simulink model "system_identification_good"  (R2024a)
settings: Solver=ode4  StartTime=0.0  StopTime=inf  FixedStep=0.002  RelTol=1e-3  EnableMultiTasking=on
undefined symbols (not defined in the file or in its folder): HIL
libraries: quarc_library x6
settings Model: ExtModeTrigDuration=10000  Creator=brusie  LastModifiedBy=brusie
settings SolverCC: AlgebraicLoopSolver=TrustRegion  PositivePriorityOrder=on
settings DataIOCC: ReturnWorkspaceOutputs=off
settings DebuggingCC: UnconnectedInputMsg=warning  UnconnectedOutputMsg=warning  UnconnectedLineMsg=warning  ArithmeticOperatorsInVariantConditions=warning
settings ModelReferenceCC: EnableRefExpFcnMdlSchedulingChecks=on
settings SFSimCC: SimUseLocalCustomCode=off  CustomCodeUndefinedFunction=UseInterfaceOnly
settings RTWCC: Description=QUARC Win64 Target Using Toolchain  SystemTargetFile=quarc_win64.tlc  TemplateMakefile=quarc_default_tmf  RTWUseLocalCustomCode=off  Toolchain=QUARC win64 | nmake (64-bit Windows)  BuildConfiguration=Faster Runs  GPUComputeCapability=3.5
settings CodeAppCC: StateflowObjectComments=on
settings STFCustomTargetCC: ConcurrentExecutionCompliant=on  SystemTargetFile=quarc_win64.tlc
settings GRTTargetCC: ParMdlRefBuildCompliant=off  CompOptLevelCompliant=off  CombineOutputUpdateFcns=off  MatFileLogging=off  CPPClassGenCompliant=off  GRTInterface=on  ExtMode=on  ExtModeMexFile=quarc_comm
settings ConfigComp: CovMetricSettings=dswe

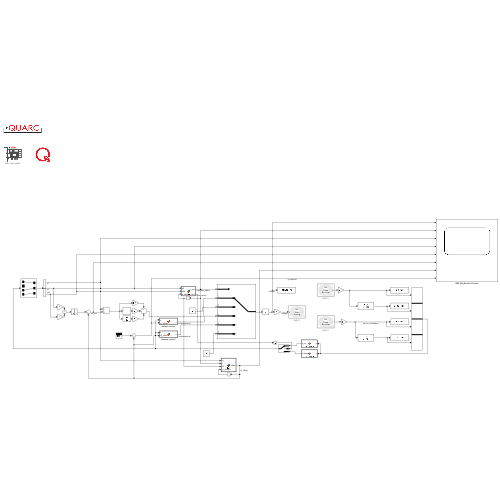
[thumbnail: Simulink's stored preview of the top-level diagram]
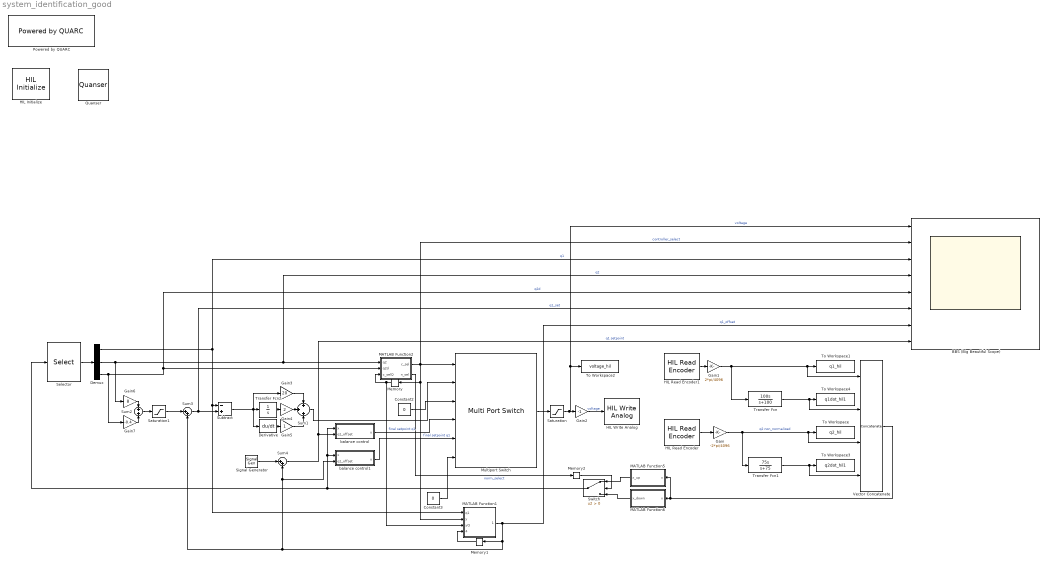
== system system_identification_good ==
  BBS (Big Beautiful Scope) : Scope  NumInputPorts=8
  Constant2 : Constant  Value=0
  Constant3 : Constant  Value=0
  Demux : Demux  Outputs=3
      settings: DisplayOption=none
  Derivative : Derivative
  Gain : Gain  Gain=-2*pi/4096
  Gain1 : Gain  Gain=2*pi/4096
  Gain2 : Gain  Gain=-1
  Gain3 : Gain  Gain=20
  Gain4 : Gain  Gain=2
  Gain5 : Gain
  Gain6 : Gain  Gain=8
  Gain7 : Gain  Gain=-0.4
  HIL Initialize : quarc_library/Data Acquisition/Generic/Configuration/HIL Initialize  object_name=HIL-1  board_type=q2_usb  board_number=0  board_options=d0=digital;d1=digital;led=auto;update_rate=normal;decimation=1  exclusive=off  active=on  hardware_clocks=[0]  clock_modes=[]  initial_clock_frequencies=[]  set_clock_params_at_start=off  set_clock_params_at_switch_in=off  set_clock_frequencies_at_start=off  set_clock_frequencies_at_switch_in=off  analog_input_channels=[0:1]  analog_input_configurations=[]  analog_input_maximums=10  analog_input_minimums=-10  set_analog_input_params_at_start=on  set_analog_input_params_at_switch_in=off  analog_output_channels=[0:1]  analog_output_maximums=10  analog_output_minimums=-10  initial_analog_outputs=[0]  final_analog_outputs=[0]  watchdog_analog_outputs=0  set_analog_output_params_at_start=on  set_analog_output_params_at_switch_in=off  set_analog_outputs_at_start=on  set_analog_outputs_at_switch_in=off  set_analog_outputs_at_terminate=on  set_analog_outputs_at_switch_out=off  set_analog_outputs_on_watchdog=off  digital_input_channels=[]  digital_output_channels=[]  digital_output_configuration=[]  initial_digital_outputs=[1]  final_digital_outputs=[1]  watchdog_digital_outputs=[1]  set_digital_output_params_at_start=off  set_digital_output_params_at_switch_in=off  set_digital_outputs_at_start=on  set_digital_outputs_at_switch_in=off  set_digital_outputs_at_terminate=on  set_digital_outputs_at_switch_out=off  set_digital_outputs_on_watchdog=off  encoder_channels=[0:1]  quadrature=[4]  encoder_filter_frequency=[]  initial_encoder_counts=[0]  set_encoder_params_at_start=on  set_encoder_params_at_switch_in=off  set_encoder_counts_at_start=on  set_encoder_counts_at_switch_in=off  pwm_channels=[]  pwm_modes=[0]  pwm_frequency=1/0.020  pwm_configuration=[]  pwm_alignment=[]  pwm_polarity=[]  pwm_leading_deadband=[]  pwm_trailing_deadband=[]  initial_pwm_outputs=[0]  final_pwm_outputs=[0]  watchdog_pwm_outputs=[0]  set_pwm_params_at_start=on  set_pwm_params_at_switch_in=off  set_pwm_outputs_at_start=on  set_pwm_outputs_at_switch_in=off  set_pwm_outputs_at_terminate=on  set_pwm_outputs_at_switch_out=off  set_pwm_outputs_on_watchdog=off  other_output_channels=[]  initial_other_outputs=[]  final_other_outputs=[]  watchdog_other_outputs=[]  set_other_outputs_at_start=off  set_other_outputs_at_switch_in=off  set_other_outputs_at_terminate=off  set_other_outputs_at_switch_out=off  set_other_outputs_on_watchdog=off
  HIL Read Encoder : quarc_library/Data Acquisition/Generic/Immediate I//O/HIL Read Encoder  object_name=HIL-1  channels=[1]  sample_time=qc_get_step_size  active=on  vector_output=off  data_type_mode=Inherit via back propagation  data_type=double
  HIL Read Encoder1 : quarc_library/Data Acquisition/Generic/Immediate I//O/HIL Read Encoder  object_name=HIL-1  channels=0  sample_time=qc_get_step_size  active=on  vector_output=off  data_type_mode=Inherit via back propagation  data_type=double
  HIL Write Analog : quarc_library/Data Acquisition/Generic/Immediate I//O/HIL Write Analog  object_name=HIL-1  channels=0  sample_time=-1  active=off  vector_input=off
  MATLAB Function1 : MATLAB Function  TreatAsAtomicUnit=on
  MATLAB Function2 : MATLAB Function  TreatAsAtomicUnit=on
  MATLAB Function5 : MATLAB Function  TreatAsAtomicUnit=on
  MATLAB Function6 : MATLAB Function  TreatAsAtomicUnit=on
  Memory : Memory
  Memory1 : Memory
  Memory2 : Memory
  Multiport Switch : MultiPortSwitch  Inputs=4  DataPortForDefault=Additional data port  SaturateOnIntegerOverflow=off  InputSameDT=off
  Powered by QUARC : quarc_library/Logos/Powered by QUARC
  Quanser : quarc_library/Logos/Quanser
  Saturation : Saturate  UpperLimit=10  LowerLimit=-10
  Saturation1 : Saturate  UpperLimit=pi/6  LowerLimit=-pi/6
  Selector : Selector  InputPortWidth=4  IndexOptions=Index vector (dialog)  Indices=[1 3 4]  OutputSizes=1
  Signal Generator : SignalGenerator  Amplitude=0  Units=rad/sec
  Subtract : Sum  Inputs=-+
  Sum1 : Sum  Inputs=+|+|+
  Sum2 : Sum
  Sum3 : Sum  Inputs=|++
  Sum4 : Sum  Inputs=|++
  Switch : Switch  Criteria=u2 > Threshold  SaturateOnIntegerOverflow=off  InputSameDT=off
  To Workspace : ToWorkspace  VariableName=q2_hil  SaveFormat=Structure With Time  SampleTime=-1
  To Workspace1 : ToWorkspace  VariableName=q1_hil  SaveFormat=Structure With Time  SampleTime=-1
  To Workspace2 : ToWorkspace  VariableName=voltage_hil  SaveFormat=Structure With Time  SampleTime=-1
  To Workspace3 : ToWorkspace  VariableName=q2dot_hil1  SaveFormat=Structure With Time  SampleTime=-1
  To Workspace4 : ToWorkspace  VariableName=q1dot_hil1  SaveFormat=Structure With Time  SampleTime=-1
  Transfer Fcn : TransferFcn  Numerator=[100 0]  Denominator=[1 100]
  Transfer Fcn1 : TransferFcn  Numerator=[75 0]  Denominator=[1 75]
  Transfer Fcn2 : TransferFcn  Denominator=[1 0]
  Vector Concatenate : Concatenate  NumInputs=4
  balance control : MATLAB Function  TreatAsAtomicUnit=on
  balance control1 : MATLAB Function  TreatAsAtomicUnit=on
  wires:
  Saturation/1 -> To Workspace2/1, BBS (Big Beautiful Scope)/1, Gain2/1  "voltage"
  Gain1/1 -> Vector Concatenate/1, To Workspace1/1, Transfer Fcn/1
  HIL Read Encoder1/1 -> Gain1/1
  HIL Read Encoder/1 -> Gain/1
  Transfer Fcn/1 -> Vector Concatenate/2, To Workspace4/1
  Transfer Fcn1/1 -> Vector Concatenate/4, To Workspace3/1
  Constant2/1 -> Multiport Switch/3
  Derivative/1 -> Gain5/1
  Transfer Fcn2/1 -> Gain4/1
  Gain3/1 -> Sum1/1
  Gain5/1 -> Sum1/3
  Gain4/1 -> Sum1/2
  Demux/3 -> Gain7/1, MATLAB Function2/2(q2d), BBS (Big Beautiful Scope)/5  "q2d"
  Gain7/1 -> Sum2/2
  Memory/1 -> MATLAB Function2/3(c_selQ), MATLAB Function1/3(yQ)
  Multiport Switch/1 -> Saturation/1
  Gain6/1 -> Sum2/1
  Gain/1 -> Vector Concatenate/3, To Workspace/1, Transfer Fcn1/1  "q2 non_normalized"
  Demux/1 -> BBS (Big Beautiful Scope)/3, MATLAB Function1/1(q1), Subtract/1  "q1"
  Selector/1 -> Demux/1
  Gain2/1 -> HIL Write Analog/1  "voltage"
  MATLAB Function1/1(q1_offset) -> Sum3/2, balance control1/2(q1_offset), Sum4/2, Memory1/1, BBS (Big Beautiful Scope)/7  "q1_offset"
  Memory1/1 -> MATLAB Function1/4(q1_offsetQ)
  Sum2/1 -> Saturation1/1
  Subtract/1 -> Derivative/1, Gain3/1, Transfer Fcn2/1
  Sum1/1 -> Multiport Switch/2
  Saturation1/1 -> Sum3/1
  Sum3/1 -> BBS (Big Beautiful Scope)/6, Subtract/2  "q1_set"
  Signal Generator/1 -> Sum4/1
  Sum4/1 -> BBS (Big Beautiful Scope)/8, balance control/2(q1_offset)  "q1 setpoint"
  MATLAB Function6/1(x_down) -> Switch/3
  MATLAB Function5/1(x_up) -> Switch/1
  Vector Concatenate/1 -> MATLAB Function5/1(x), MATLAB Function6/1(x)
  MATLAB Function2/2(n_sel) -> Memory2/1  "norm_select"
  Switch/1 -> Selector/1, balance control/1(x), balance control1/1(x)
  Demux/2 -> Gain6/1, BBS (Big Beautiful Scope)/4, MATLAB Function2/1(q2)  "q2"
  Memory2/1 -> Switch/2
  MATLAB Function2/1(c_sel) -> Multiport Switch/1, BBS (Big Beautiful Scope)/2, Memory/1, MATLAB Function1/2(y)  "controller_select"
  balance control/1(u) -> Multiport Switch/4  "final setpoint q1"
  Constant3/1 -> Multiport Switch/6
  balance control1/1(u) -> Multiport Switch/5  "final setpoint q1"

== matlab function system_identification_good/MATLAB Function1 ==
  data: q1 input; y input; q1_offset output; yQ input; q1_offsetQ input
function q1_offset = fcn(q1, y, yQ, q1_offsetQ)

if (yQ == 2 || yQ == 4) && y == 1
    q1_offset = q1;
else
    q1_offset = q1_offsetQ;
end
end

== matlab function system_identification_good/balance control ==
  data: x input; u output; q1_offset input
function u = K(x, q1_offset)
    q1 = x(1)-q1_offset;
    xp = [q1, x(2), x(3), x(4)]';
    k = [-0.5376	-0.9225	-12.0174	-1.3906];
    u = -k*xp;
end

== matlab function system_identification_good/MATLAB Function2 ==
  data: q2 input; q2d input; c_sel output; c_selQ input; n_sel output
function [c_sel,n_sel] = fcn(q2, q2d, c_selQ)

%q2 = x(3);


if c_selQ == 1
    if abs(q2) > 5*pi/6
        c_sel = 3;
    else
        c_sel = c_selQ;
    end
elseif c_selQ == 2
    if abs(q2) < pi/3
        c_sel = 4;  %%% eventuallc_sel replace this with 4
    else
        c_sel = c_selQ;
    end
elseif c_selQ == 3
    if abs(q2) > pi/6
        c_sel = 2;
    else
        c_sel = c_selQ;
    end
elseif c_selQ == 4
    if abs(q2d) < 13 || abs(q2) < pi/8 %&& abs(q2d) < 0.1
        c_sel = 1;
    else
        c_sel = c_selQ;
    end
else
    c_sel = 2;
end



if c_sel == 1
    n_sel = 0;
elseif c_sel == 2
    n_sel = 0;
elseif c_sel == 3
    n_sel = 1;
elseif c_sel == 4
    n_sel = 0;
else
    n_sel = 0;
end

end

== matlab function system_identification_good/balance control1 ==
  data: x input; u output; q1_offset input
function u = K(x, q1_offset)
    q1 = x(1)-q1_offset;
    xp = [q1, x(2), x(3), x(4)]';
    k = [-0.0131	-0.5224	-5.1436	-0.3850];
    u = k*xp; % positive because renormalization had that happen
end

== matlab function system_identification_good/MATLAB Function5 ==
  data: x input; x_up output
function x_up = normalize(x)
    q2 = x(3)+pi;
    x_up = [x(1), x(2), atan2(sin(q2),cos(q2)), x(4)]';
end

== matlab function system_identification_good/MATLAB Function6 ==
  data: x input; x_down output
function x_down = normalize(x)
    q2 = x(3);
    x_down = [x(1), x(2), atan2(sin(q2),cos(q2)), x(4)]';
end
